simulink model "ThreePhase_Inverter_SVM"  (R2023a)
settings: Solver=ode23t  StartTime=0.0  StopTime=0.05  MaxStep=1e-4  RelTol=1e-3
libraries: spsMosfetLib x12, simulink x4, spsSeriesRLCBranchLib x3, spsDCVoltageSourceLib x2, spsGroundLib x2, spsThreePhaseVIMeasurementLib x2, spspowerguiLib x2, spsFundamentalPLLDrivenLib x1, spsPLLLib x1, spsThreePhaseSeriesRLCBranchLib x1
settings Model: Creator=Alielden  LastModifiedBy=Alielden
settings DataIOCC: SaveState=on  SignalLogging=off  DSMLogging=off  ReturnWorkspaceOutputs=off  LoggingToFile=on

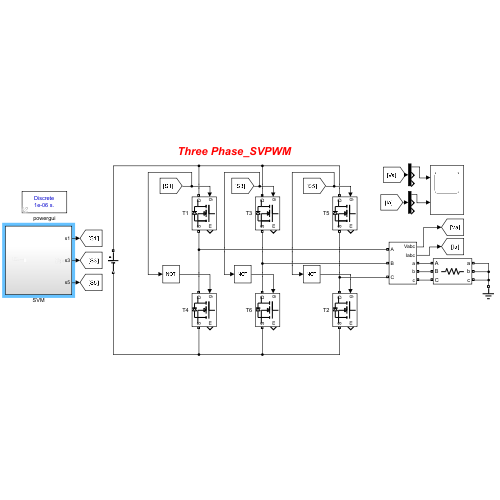
[thumbnail: Simulink's stored preview of the top-level diagram]
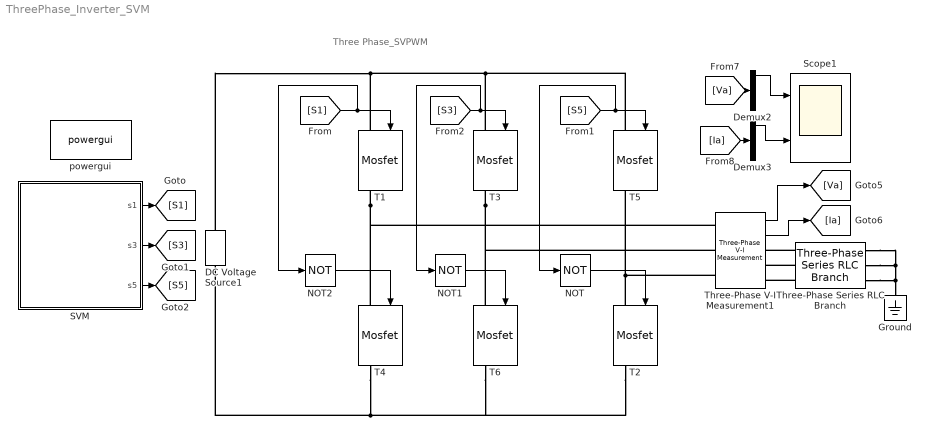
== system ThreePhase_Inverter_SVM ==
  note: Three Phase_SVPWM
  DC Voltage Source1 : spsDCVoltageSourceLib/DC Voltage Source  Amplitude=320  Measurements=None
  Demux2 : Demux  Outputs=3
  Demux3 : Demux  Outputs=3
  Ground : spsGroundLib/Ground  LConnTagsString=a
  NOT : Logic  Operator=NOT  AllPortsSameDT=off  OutDataTypeStr=boolean
  NOT1 : Logic  Operator=NOT  AllPortsSameDT=off  OutDataTypeStr=boolean
  NOT2 : Logic  Operator=NOT  AllPortsSameDT=off  OutDataTypeStr=boolean
  SVM : Subsystem
  Scope1 : Scope  NumInputPorts=2
  T{1..6} (6 alike) : spsMosfetLib/Mosfet  Ron=0.1  Lon=0  Rd=0.01  Vfd=0  IC=0  Rs=1e5  Cs=inf  Measurements=on
  Three-Phase Series RLC Branch : spsThreePhaseSeriesRLCBranchLib/Three-Phase Series RLC Branch  LConnTagsString=A|B|C  RConnTagsString=A|B|C  BranchType=R  Resistance=10  Inductance=1e-3  Capacitance=1e-6  Measurements=None
  Three-Phase V-I Measurement1 : spsThreePhaseVIMeasurementLib/Three-Phase V-I Measurement  VoltageMeasurement=phase-to-ground  SetLabelV=off  LabelV=Van  Vpu=off  VpuLL=off  CurrentMeasurement=yes  SetLabelI=off  LabelI=Iabc  Ipu=off  Pbase=100e6  Vbase=500e3  OutputType=Complex  PhasorSimulation=off  PSBequivalent=0
  powergui : spspowerguiLib/powergui  Priority=1  SimulationMode=Discrete  SampleTime=1e-6  frequency=60  Iterations=50  frequencyindice=0  Pbase=100e6  ErrMax=1e-4  UnitsV=kV  UnitsW=MW  buscounter=0  FunctionMessages=off  echomessages=off  EnableUseOfTLC=off  CurrentSourceSwitches=off  DisableSnubberDevices=off  DisableRonSwitches=off  DisableVfSwitches=off  DisplayEquations=off  AutomaticDiscreteSolvers=off  SolverType=Tustin/Backward Euler (TBE)  Interpol=off  ExternalGateDelay=off  methode=off  Ts=100  x0status=blocks  SPID=on  SwTol=0  HookPort=off  NonlinearTolerance=1e-4  nMaxIteration=100  ContinueOnMaxIteration=off  RestoreLinks=warning  ResistiveCurrentMeasurement=off  Frange=[0:2:500]  Ylog=off  Xlog=on  ShowGrid=off  save=off  variable=ZData  structure=0  ZoomFFT=off  StartTime=0.0  cycles=1  DisplayStyle=1  fundamental=60  FreqAxis=off  MaxFrequency=1000  frequencyindicesteady=1  RmsSteady=1  display=off
  wires:
  SVM/2(s3) -> [S3]
  NOT2/1 -> T4/1
  [S3] -> NOT1/1, T3/1
  SVM/3(s5) -> [S5]
  SVM/1(s1) -> [S1]
  NOT/1 -> T2/1
  [S5] -> NOT/1, T5/1
  NOT1/1 -> T6/1
  [S1] -> NOT2/1, T1/1
  Demux2/1 -> Scope1/1
  Demux3/1 -> Scope1/2
  [Va] -> Demux2/1
  [Ia] -> Demux3/1
  Three-Phase V-I Measurement1/2 -> [Ia]
  Three-Phase V-I Measurement1/1 -> [Va]
  connections:
  Three-Phase V-I Measurement1/LConn3 -- T5/RConn1 -- T2/LConn1
  T1/RConn1 -- T4/LConn1 -- Three-Phase V-I Measurement1/LConn1
  T3/LConn1 -- T5/LConn1 -- DC Voltage Source1/RConn1 -- T1/LConn1
  T3/RConn1 -- T6/LConn1 -- Three-Phase V-I Measurement1/LConn2
  T4/RConn1 -- DC Voltage Source1/LConn1 -- T2/RConn1 -- T6/RConn1
  Three-Phase Series RLC Branch/LConn2 -- Three-Phase V-I Measurement1/RConn2
  Three-Phase Series RLC Branch/LConn1 -- Three-Phase V-I Measurement1/RConn1
  Three-Phase Series RLC Branch/LConn3 -- Three-Phase V-I Measurement1/RConn3
  Three-Phase Series RLC Branch/RConn1 -- Three-Phase Series RLC Branch/RConn2 -- Three-Phase Series RLC Branch/RConn3 -- Ground/LConn1

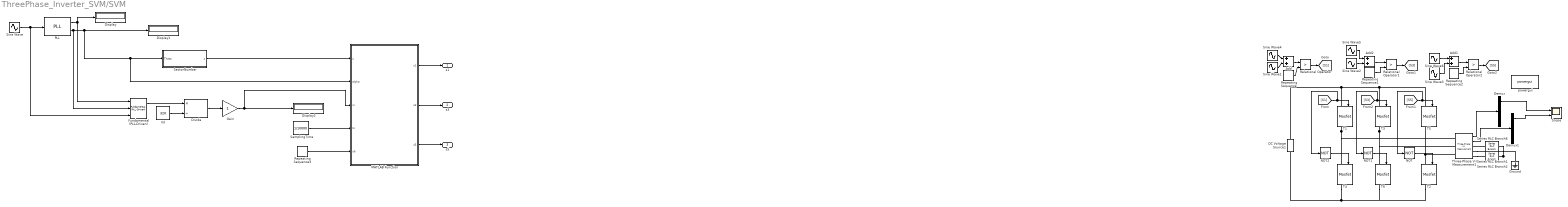
== system ThreePhase_Inverter_SVM/SVM ==
  Add : Sum
  Add1 : Sum
  Add2 : Sum
  DC Voltage Source1 : spsDCVoltageSourceLib/DC Voltage Source  Amplitude=100  Measurements=None
  Demux : Demux  Outputs=3
  Demux1 : Demux  Outputs=3
  Display : Display
  Display1 : Display
  Display2 : Display
  Divide : Product  Inputs=*/
  Fundamental (PLL-Driven) : spsFundamentalPLLDrivenLib/Fundamental (PLL-Driven)  Finit=60  Fmin=45  InInit=[1, 0]  Ts=0
      settings: LibrarySourceBlock=|
      | sps_lib/Sensors and Measurements/Fundamental
      | (PLL-Driven)
  Gain : Gain
  Ground : spsGroundLib/Ground  LConnTagsString=a
  MATLAB Function : MATLAB Function  TreatAsAtomicUnit=on
  NOT : Logic  Operator=NOT  AllPortsSameDT=off  OutDataTypeStr=boolean
  NOT1 : Logic  Operator=NOT  AllPortsSameDT=off  OutDataTypeStr=boolean
  NOT2 : Logic  Operator=NOT  AllPortsSameDT=off  OutDataTypeStr=boolean
  PLL : spsPLLLib/PLL  Fmin=45  Par_Init=[0, 50]  ParK=[180, 3200, 1]  TcD=1e-4  MaxRateChangeFreq=15  FilterCutOffFreq=25  Ts=0  AGC=on
      settings: LibrarySourceBlock=sps_lib/Control/PLL
  Relational Operator : RelationalOperator  Operator=>  OutDataTypeStr=boolean  RndMeth=Simplest  InputSameDT=off
  Relational Operator1 : RelationalOperator  Operator=>  OutDataTypeStr=boolean  RndMeth=Simplest  InputSameDT=off
  Relational Operator2 : RelationalOperator  Operator=>  OutDataTypeStr=boolean  RndMeth=Simplest  InputSameDT=off
  Repeating Sequence : simulink/Sources/Repeating Sequence  rep_seq_t="[0 (1/5000)/4  (1/5000)/2  3*(1/5000)/4  (1/5000)]"  rep_seq_y=[0 1 0 -1 0]
  Repeating Sequence1 : simulink/Sources/Repeating Sequence  rep_seq_t="[0 (1/5000)/4  (1/5000)/2  3*(1/5000)/4  (1/5000)]"  rep_seq_y=[0 1 0 -1 0]
  Repeating Sequence2 : simulink/Sources/Repeating Sequence  rep_seq_t="[0 (1/5000)/4  (1/5000)/2  3*(1/5000)/4  (1/5000)]"  rep_seq_y=[0 1 0 -1 0]
  Repeating Sequence3 : simulink/Sources/Repeating Sequence  rep_seq_t=[0 (1/10000)]  rep_seq_y=[0 (1/10000)]
  SamplingTime : Constant  Value=1/10000
  Scope : Scope  NumInputPorts=2
  SectorNumber : Subsystem
  Series RLC Branch1 : spsSeriesRLCBranchLib/Series RLC Branch  LConnTagsString=__new0  RConnTagsString=__new0  BranchType=R  Resistance=10  Inductance=1e-3  SetiL0=off  InitialCurrent=0  Capacitance=1e-6  Setx0=off  InitialVoltage=0  Measurements=None
  Series RLC Branch2 : spsSeriesRLCBranchLib/Series RLC Branch  LConnTagsString=__new0  RConnTagsString=__new0  BranchType=R  Resistance=10  Inductance=1e-3  SetiL0=off  InitialCurrent=0  Capacitance=1e-6  Setx0=off  InitialVoltage=0  Measurements=None
  Series RLC Branch6 : spsSeriesRLCBranchLib/Series RLC Branch  LConnTagsString=__new0  RConnTagsString=__new0  BranchType=R  Resistance=10  Inductance=1e-3  SetiL0=off  InitialCurrent=0  Capacitance=1e-6  Setx0=off  InitialVoltage=0  Measurements=None
  Sine Wave : Sin  Amplitude=220*sqrt(2)  Frequency=100*pi  SampleTime=1/10000
  Sine Wave1 : Sin  Amplitude=1.15  Frequency=100*pi  SampleTime=0
  Sine Wave2 : Sin  Amplitude=1.15  Frequency=100*pi  Phase=120*pi/180  SampleTime=0
  Sine Wave3 : Sin  Amplitude=1.15  Frequency=100*pi  Phase=240*pi/180  SampleTime=0
  Sine Wave4 : Sin  Amplitude=0.19  Frequency=100*pi*3  SampleTime=0
  Sine Wave5 : Sin  Amplitude=0.19  Frequency=100*pi*3  Phase=120*pi/180  SampleTime=0
  Sine Wave6 : Sin  Amplitude=0.19  Frequency=100*pi*3  Phase=240*pi/180  SampleTime=0
  T{1..6} (6 alike) : spsMosfetLib/Mosfet  Ron=0.1  Lon=0  Rd=0.01  Vfd=0  IC=0  Rs=1e5  Cs=inf  Measurements=on
  Three-Phase V-I Measurement1 : spsThreePhaseVIMeasurementLib/Three-Phase V-I Measurement  VoltageMeasurement=phase-to-ground  SetLabelV=off  LabelV=Van  Vpu=off  VpuLL=off  CurrentMeasurement=yes  SetLabelI=off  LabelI=Iabc  Ipu=off  Pbase=100e6  Vbase=500e3  OutputType=Complex  PhasorSimulation=off  PSBequivalent=0
  Vd : Constant  Value=320
  powergui : spspowerguiLib/powergui  Priority=1  SimulationMode=Discrete  SampleTime=1e-6  frequency=60  Iterations=50  frequencyindice=0  Pbase=100e6  ErrMax=1e-4  UnitsV=kV  UnitsW=MW  buscounter=0  FunctionMessages=off  echomessages=off  EnableUseOfTLC=off  CurrentSourceSwitches=off  DisableSnubberDevices=off  DisableRonSwitches=off  DisableVfSwitches=off  DisplayEquations=off  AutomaticDiscreteSolvers=off  SolverType=Tustin/Backward Euler (TBE)  Interpol=off  ExternalGateDelay=off  methode=off  Ts=100  x0status=blocks  SPID=on  SwTol=0  HookPort=off  NonlinearTolerance=1e-4  nMaxIteration=100  ContinueOnMaxIteration=off  RestoreLinks=warning  ResistiveCurrentMeasurement=off  Frange=[0:2:500]  Ylog=off  Xlog=on  ShowGrid=off  save=off  variable=ZData  structure=0  ZoomFFT=off  StartTime=0.0  cycles=1  DisplayStyle=1  fundamental=60  FreqAxis=off  MaxFrequency=1000  frequencyindicesteady=1  RmsSteady=1  display=off
  s1 : Outport
  s3 : Outport  Port=2
  s5 : Outport  Port=3
  wires:
  MATLAB Function/1(s1) -> s1/1
  Sine Wave/1 -> Fundamental (PLL-Driven)/3, PLL/1
  PLL/1 -> Fundamental (PLL-Driven)/1, Display/1
  Add/1 -> Relational Operator/1
  Sine Wave1/1 -> Add/2
  Sine Wave4/1 -> Add/1
  Sine Wave2/1 -> Add2/2
  Add2/1 -> Relational Operator1/1
  Relational Operator1/1 -> [S3]
  Demux/1 -> Scope/1
  NOT2/1 -> T4/1
  [S3] -> NOT1/1, T3/1
  Repeating Sequence1/1 -> Relational Operator1/2
  Sine Wave6/1 -> Add1/1
  Repeating Sequence/1 -> Relational Operator/2
  Relational Operator2/1 -> [S5]
  Sine Wave5/1 -> Add2/1
  Relational Operator/1 -> [S1]
  NOT/1 -> T2/1
  Three-Phase V-I Measurement1/1 -> Demux/1
  Sine Wave3/1 -> Add1/2
  Demux1/1 -> Scope/2
  [S5] -> NOT/1, T5/1
  Repeating Sequence2/1 -> Relational Operator2/2
  Three-Phase V-I Measurement1/2 -> Demux1/1
  NOT1/1 -> T6/1
  [S1] -> NOT2/1, T1/1
  Add1/1 -> Relational Operator2/1
  PLL/2 -> Fundamental (PLL-Driven)/2, MATLAB Function/2(alpha), SectorNumber/1(Theta), Display1/1
  Divide/1 -> Gain/1
  Fundamental (PLL-Driven)/1 -> Divide/1
  Vd/1 -> Divide/2
  Gain/1 -> MATLAB Function/3(m), Display2/1
  SectorNumber/1(s) -> MATLAB Function/1(s)
  SamplingTime/1 -> MATLAB Function/4(ts)
  Repeating Sequence3/1 -> MATLAB Function/5(clk)
  MATLAB Function/2(s3) -> s3/1
  MATLAB Function/3(s5) -> s5/1
  connections:
  Three-Phase V-I Measurement1/LConn3 -- T5/RConn1 -- T2/LConn1
  T1/RConn1 -- T4/LConn1 -- Three-Phase V-I Measurement1/LConn1
  T3/LConn1 -- T5/LConn1 -- DC Voltage Source1/RConn1 -- T1/LConn1
  T3/RConn1 -- T6/LConn1 -- Three-Phase V-I Measurement1/LConn2
  T4/RConn1 -- DC Voltage Source1/LConn1 -- T2/RConn1 -- T6/RConn1
  Series RLC Branch2/RConn1 -- Series RLC Branch6/RConn1 -- Ground/LConn1 -- Series RLC Branch1/RConn1
  Three-Phase V-I Measurement1/RConn2 -- Series RLC Branch1/LConn1
  Series RLC Branch6/LConn1 -- Three-Phase V-I Measurement1/RConn1
  Three-Phase V-I Measurement1/RConn3 -- Series RLC Branch2/LConn1

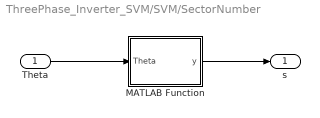
== system ThreePhase_Inverter_SVM/SVM/SectorNumber ==
  Theta : Inport
  MATLAB Function : MATLAB Function  TreatAsAtomicUnit=on
  s : Outport
  wires:
  Theta/1 -> MATLAB Function/1(Theta)
  MATLAB Function/1(y) -> s/1

== matlab function ThreePhase_Inverter_SVM/SVM/MATLAB Function ==
  data: s input; s1 output; alpha input; m input; ts input; clk input; s3 output; s5 output
function [s1,s3,s5] = fcn(s,alpha,m,ts,clk)

ta = ts * m * sin(pi/3-(alpha-(s-1)*pi/3));
tb = ts * m * sin(alpha-(s-1)*pi/3);
t0=ts - (ta+tb) ;

switch(s)
    case(1)
        if( (clk>t0/4)  &&  (clk<(t0/4+ta/2+tb/2+t0/2+tb/2+ta/2)) )
            s1=1;
        else
            s1=0;
        end
        if( (clk>(t0/4+ta/2))  &&  (clk<(t0/4+ta/2+tb/2+t0/2+tb/2)) )
            s3=1;
        else
            s3=0;
        end
        if( (clk>(t0/4+ta/2+tb/2))  &&  (clk<(t0/4+ta/2+tb/2+t0/2)) )
            s5=1;
        else
            s5=0;
        end

    case(2)
        if( (clk>t0/4)  &&  (clk<(t0/4+ta/2+tb/2+t0/2+tb/2+ta/2)) )
            s3=1;
        else
            s3=0;
        end
        if( (clk>(t0/4+ta/2))  &&  (clk<(t0/4+ta/2+tb/2+t0/2+tb/2)) )
            s1=1;
        else
            s1=0;
        end
        if( (clk>(t0/4+ta/2+tb/2))  &&  (clk<(t0/4+ta/2+tb/2+t0/2)) )
            s5=1;
        else
            s5=0;
        end

    case(3)
        if( (clk>t0/4)  &&  (clk<(t0/4+ta/2+tb/2+t0/2+tb/2+ta/2)) )
            s3=1;
        else
            s3=0;
        end
        if( (clk>(t0/4+ta/2))  &&  (clk<(t0/4+ta/2+tb/2+t0/2+tb/2)) )
            s5=1;
        else
            s5=0;
        end
        if( (clk>(t0/4+ta/2+tb/2))  &&  (clk<(t0/4+ta/2+tb/2+t0/2)) )
            s1=1;
        else
            s1=0;
        end

    case(4)
        if( (clk>t0/4)  &&  (clk<(t0/4+ta/2+tb/2+t0/2+tb/2+ta/2)) )
            s5=1;
        else
            s5=0;
        end
        if( (clk>(t0/4+ta/2))  &&  (clk<(t0/4+ta/2+tb/2+t0/2+tb/2)) )
            s3=1;
        else
            s3=0;
        end
        if( (clk>(t0/4+ta/2+tb/2))  &&  (clk<(t0/4+ta/2+tb/2+t0/2)) )
            s1=1;
        else
            s1=0;
        end

    case(5)
        if( (clk>t0/4)  &&  (clk<(t0/4+ta/2+tb/2+t0/2+tb/2+ta/2)) )
            s5=1;
        else
            s5=0;
        end
        if( (clk>(t0/4+ta/2))  &&  (clk<(t0/4+ta/2+tb/2+t0/2+tb/2)) )
            s1=1;
        else
            s1=0;
        end
        if( (clk>(t0/4+ta/2+tb/2))  &&  (clk<(t0/4+ta/2+tb/2+t0/2)) )
            s3=1;
        else
            s3=0;
        end

    case(6)
        if( (clk>t0/4)  &&  (clk<(t0/4+ta/2+tb/2+t0/2+tb/2+ta/2)) )
            s1=1;
        else
            s1=0;
        end
        if( (clk>(t0/4+ta/2))  &&  (clk<(t0/4+ta/2+tb/2+t0/2+tb/2)) )
            s5=1;
        else
            s5=0;
        end
        if( (clk>(t0/4+ta/2+tb/2))  &&  (clk<(t0/4+ta/2+tb/2+t0/2)) )
            s3=1;
        else
            s3=0;
        end

    otherwise
        s1=0;
        s3=0;
        s5=0;
end

== matlab function ThreePhase_Inverter_SVM/SVM/SectorNumber/MATLAB Function ==
  data: Theta input; y output
function y = fcn(Theta)
%#eml
if( ( Theta >= 0 ) && ( Theta <= (pi/3) ) )
    u = 1 ;

elseif( ( Theta > (pi/3) ) && ( Theta <= (2*pi/3) ) )
    u = 2 ;

elseif( ( Theta > (2*pi/3) ) && ( Theta <= (pi) ) )
    u = 3 ;

elseif( ( Theta > (pi) ) && ( Theta <= (4*pi/3) ) )
    u = 4 ;

elseif( ( Theta > (4*pi/3) ) && ( Theta <= (5*pi/3) ) )
    u = 5 ;

else
    u = 6 ;

end
y=u;
